simulink model "SildeModel_control_compare"  (R2022b)
settings: Solver=ode4  StartTime=0.0  StopTime=t_total  FixedStep=sim_dt  RelTol=1e-3  EnableMultiTasking=on
InitFcn:
  | InitialCondition
values from neighbouring files (symbols this model uses):
  I_B = diag([200, 250, 300])    [InitialCondition.m]
  lambda_max_J = max(eig(I_B))    [InitialCondition.m]
  mrp0 = [0.2, 0.3, -0.3]    [InitialCondition.m]
  MRP_REAL0 = MRP_REAL0'    [InitialCondition.m]
  mrpf = [0 0 0]'    [InitialCondition.m]
  sim_dt = 0.01    [InitialCondition.m]
  Tau_SEQ = [Tau_SEQ;   Tau_EXT]    [InitialCondition.m]
  w0 = w0(:)    [Gauss_opt_mrp.m]    (also in InitialCondition.m = [0; 0; 0])
settings Model: Creator=Administrator  LastModifiedBy=33592
settings DataIOCC: ExternalInput=[t, y]  LimitDataPoints=on  MaxDataPoints=15000  ReturnWorkspaceOutputs=off
settings OptimizationCC: LifeSpan=inf
settings DebuggingCC: MultiTaskCondExecSysMsg=warning  MultiTaskRateTransMsg=warning  UnconnectedInputMsg=warning  UnconnectedOutputMsg=warning  UnconnectedLineMsg=warning  AllowSymbolicDim=off  SFUnexpectedBacktrackingDiag=warning  SFNoUnconditionalDefaultTransitionDiag=warning  SFExecutionAtInitializationDiag=none  SFMachineParentedDataDiag=warning  ArithmeticOperatorsInVariantConditions=warning
settings ModelReferenceCC: EnableRefExpFcnMdlSchedulingChecks=on  PropagateSignalLabelsOutOfModel=off
settings SFSimCC: SimUseLocalCustomCode=off  CustomCodeUndefinedFunction=UseInterfaceOnly
settings RTWCC: RTWUseLocalCustomCode=off
settings CodeAppCC: StateflowObjectComments=on
settings GRTTargetCC: TargetLangStandard=C89/C90 (ANSI)
settings ConfigComp: CovMetricSettings=dw  CovSaveCumulativeToWorkspaceVar=on  CovSaveSingleToWorkspaceVar=on  CovExternalEMLEnable=off

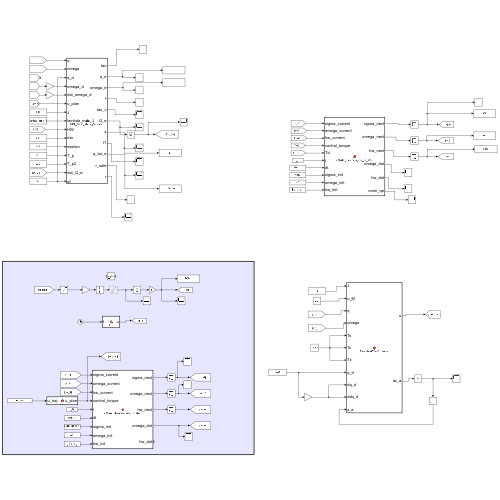
[thumbnail: Simulink's stored preview of the top-level diagram]
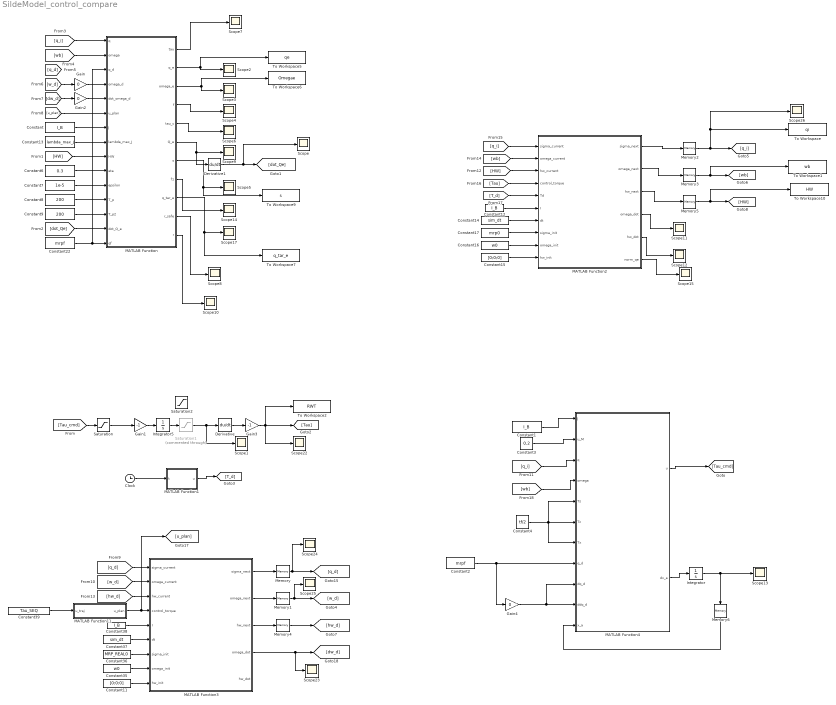
== system SildeModel_control_compare ==
  Clock : Clock
  Constant{,1,12,38} (4 alike) : Constant  Value=I_B
  Constant11 : Constant  Value=[0;0;0]
  Constant13 : Constant  Value=lambda_max_J
  Constant14 : Constant  Value=sim_dt
  Constant15 : Constant  Value=[0;0;0]
  Constant16 : Constant  Value=w0
  Constant17 : Constant  Value=mrp0
  Constant2 : Constant  Value=mrpf
  Constant22 : Constant  Value=mrpf
  Constant3 : Constant  Value=0.2
  Constant35 : Constant  Value=w0
  Constant36 : Constant  Value=MRP_REAL0
  Constant37 : Constant  Value=sim_dt
  Constant39 : Constant  Value=Tau_SEQ
  Constant4 : Constant  Value=tf/2
  Constant6 : Constant  Value=0.3
  Constant7 : Constant  Value=1e-5
  Constant8 : Constant  Value=200
  Constant9 : Constant  Value=200
  Derivative : Derivative
  Derivative1 : Derivative
  Gain : Gain  Gain=0
  Gain1 : Gain  Gain=-1
  Gain2 : Gain  Gain=0
  Gain3 : Gain  Gain=-1
  Gain4 : Gain  Gain=0
  Integrator : Integrator
  Integrator5 : Integrator
  MATLAB Function : MATLAB Function  TreatAsAtomicUnit=on
  MATLAB Function1 : MATLAB Function  TreatAsAtomicUnit=on
  MATLAB Function11 : MATLAB Function  TreatAsAtomicUnit=on
  MATLAB Function2 : MATLAB Function  TreatAsAtomicUnit=on
  MATLAB Function3 : MATLAB Function  TreatAsAtomicUnit=on
  MATLAB Function4 : MATLAB Function  TreatAsAtomicUnit=on
  Memory{,1..6} (7 alike) : Memory
  Saturation : Saturate  UpperLimit=0.2  LowerLimit=-0.2
  Saturation1 : Saturate  Commented=through  UpperLimit=4  LowerLimit=-4
  Saturation2 : Saturate  UpperLimit=4  LowerLimit=-4
  Scope{,1..15,17,22..26} (22 alike) : Scope
  To Workspace : ToWorkspace  VariableName=qi  SampleTime=-1
  To Workspace1 : ToWorkspace  VariableName=wb  SampleTime=-1
  To Workspace10 : ToWorkspace  VariableName=HW  SampleTime=-1
  To Workspace2 : ToWorkspace  VariableName=RWT  SampleTime=-1
  To Workspace5 : ToWorkspace  VariableName=qe  SampleTime=-1
  To Workspace6 : ToWorkspace  VariableName=Omegae  SampleTime=-1
  To Workspace7 : ToWorkspace  VariableName=q_tar_e  SampleTime=-1
  To Workspace9 : ToWorkspace  VariableName=s  SampleTime=-1
  wires:
  [q_i] -> MATLAB Function/1(q)
  [wb] -> MATLAB Function/2(omega)
  Constant/1 -> MATLAB Function/7(J)
  MATLAB Function/2(q_e) -> Scope2/1, To Workspace5/1
  Constant6/1 -> MATLAB Function/10(eta)
  Constant7/1 -> MATLAB Function/11(epsilon)
  Constant8/1 -> MATLAB Function/12(T_p)
  Constant9/1 -> MATLAB Function/13(T_p2)
  MATLAB Function/3(omega_e) -> Scope3/1, To Workspace6/1
  MATLAB Function/4(f) -> Scope4/1
  Constant13/1 -> MATLAB Function/8(lambda_max_J)
  MATLAB Function/7(s) -> To Workspace9/1, Scope5/1
  MATLAB Function/5(tau_c) -> Scope6/1
  MATLAB Function/6(Q_e) -> Derivative1/1, Scope9/1
  Clock/1 -> MATLAB Function1/1(t)
  MATLAB Function1/1(u) -> [T_d]
  MATLAB Function/8(f1) -> Scope14/1
  Constant22/1 -> MATLAB Function/3(q_d), MATLAB Function/15(qf)
  MATLAB Function/9(q_tar_e) -> To Workspace7/1, Scope17/1
  Gain1/1 -> Integrator5/1
  Constant35/1 -> MATLAB Function3/8(omega_init)
  Constant36/1 -> MATLAB Function3/7(sigma_init)
  Constant37/1 -> MATLAB Function3/6(dt)
  Constant38/1 -> MATLAB Function3/5(I)
  Constant39/1 -> MATLAB Function11/1(u_traj)
  MATLAB Function11/1(u_plan) -> [u_plan], MATLAB Function3/4(control_torque)
  MATLAB Function3/1(sigma_next) -> Memory/1
  Memory/1 -> [q_d], Scope24/1
  MATLAB Function3/2(omega_next) -> Memory1/1
  Memory1/1 -> [w_d], Scope25/1
  MATLAB Function3/4(omega_dot) -> Scope23/1, [dw_d]
  MATLAB Function3/3(hw_next) -> Memory4/1
  Memory4/1 -> [hw_d]
  [q_d] -> MATLAB Function3/1(sigma_current)
  [w_d] -> MATLAB Function3/2(omega_current)
  [hw_d] -> MATLAB Function3/3(hw_current)
  Constant11/1 -> MATLAB Function3/9(hw_init)
  MATLAB Function2/1(sigma_next) -> Memory2/1
  Memory3/1 -> To Workspace1/1, [wb]
  Memory2/1 -> [q_i], To Workspace/1, Scope26/1
  MATLAB Function2/2(omega_next) -> Memory3/1
  MATLAB Function2/3(hw_next) -> Memory5/1
  MATLAB Function2/4(omega_dot) -> Scope11/1
  MATLAB Function2/5(hw_dot) -> Scope12/1
  Memory5/1 -> To Workspace10/1, [HW]
  [HW] -> MATLAB Function2/3(hw_current)
  [wb] -> MATLAB Function2/2(omega_current)
  [q_i] -> MATLAB Function2/1(sigma_current)
  [Tau] -> MATLAB Function2/4(control_torque)
  [T_d] -> MATLAB Function2/5(Td)
  Constant12/1 -> MATLAB Function2/6(I)
  Constant14/1 -> MATLAB Function2/7(dt)
  Constant17/1 -> MATLAB Function2/8(sigma_init)
  Constant16/1 -> MATLAB Function2/9(omega_init)
  Constant15/1 -> MATLAB Function2/10(hw_init)
  [HW] -> MATLAB Function/9(HW)
  Derivative/1 -> Gain3/1
  Gain3/1 -> [Tau], To Workspace2/1, Scope22/1
  [u_plan] -> MATLAB Function/6(u_plan)
  [Tau_cmd] -> Saturation/1
  Saturation/1 -> Gain1/1
  Derivative1/1 -> Scope/1, [dot_Qe]
  [dot_Qe] -> MATLAB Function/14(dot_Q_e)
  MATLAB Function/10(r_safe) -> Scope8/1
  MATLAB Function/11(r) -> Scope10/1
  MATLAB Function/1(tau) -> Scope7/1
  [w_d] -> Gain/1
  [dw_d] -> Gain2/1
  Gain/1 -> MATLAB Function/4(omega_d)
  Gain2/1 -> MATLAB Function/5(dot_omega_d)
  Integrator5/1 -> Saturation1/1
  Saturation1/1 -> Scope1/1, Derivative/1
  Constant1/1 -> MATLAB Function4/1(J)
  [q_i] -> MATLAB Function4/3(q)
  [wb] -> MATLAB Function4/4(omega)
  Constant2/1 -> MATLAB Function4/8(q_d), Gain4/1
  Gain4/1 -> MATLAB Function4/9(dq_d), MATLAB Function4/10(ddq_d)
  MATLAB Function4/2(dx_a) -> Integrator/1
  Integrator/1 -> Scope13/1, Memory6/1
  Memory6/1 -> MATLAB Function4/11(x_a)
  MATLAB Function4/1(u) -> [Tau_cmd]
  Constant3/1 -> MATLAB Function4/2(u_M)
  MATLAB Function2/6(norm_qe) -> Scope15/1
  Constant4/1 -> MATLAB Function4/7(Tx), MATLAB Function4/5(Ts), MATLAB Function4/6(Tc)

== matlab function SildeModel_control_compare/MATLAB Function4 ==
  data: J input; u_M input; u output size=[3,1]; q input size=[3,1]; omega input size=[3,1]; Ts input; Tc input; Tx input; q_d input size=[3,1]; dq_d input size=[3,1]; ddq_d input size=[3,1]; x_a input size=[3,1]; dx_a output size=[3,1]
function [u, dx_a] = PrescribedTimeController(J,u_M,q, omega,Ts,Tc,Tx, q_d, dq_d, ddq_d, x_a)
    % 基于 "Distributed Prescribed-Time Attitude Coordination..." 论文设计的单航天器控制器
    % 包含预设时间收敛 (Prescribed-Time) 和 输入抗饱和 (Input Saturation)

    %% 1. 物理参数与控制器增益 (需根据实际卫星调整)
    % 惯量矩阵 [cite: 649] (示例值，请替换为真实值)
    
    

    
    % 幂次参数 (0 < v < 0.5)
    v1 = 0.1; % [cite: 242]
    v2 = 0.1; % [cite: 357]
    
    % 增益系数
    k  = 0.01;   % 滑模面增益 [cite: 235]
    k1 = 0.01;   % 控制律增益 [cite: 357]
    k2 = 40;   % 抗饱和增益 [cite: 360]
    c  = 0.01;   % 鲁棒项增益 [cite: 351]
    zeta = 0.05; % 避免抖动的平滑参数 

    %% 2. 运动学与动力学辅助计算
    % 计算 T(q) 矩阵 [cite: 83]
    q_sq = q' * q;
    I3 = eye(3);
    q_cross = [0, -q(3), q(2); q(3), 0, -q(1); -q(2), q(1), 0]; % [cite: 89]
    T_mat = 0.5 * (0.5 * (1 - q_sq) * I3 + q_cross + q * q');
    
    % 计算姿态变化率 x2 = dq (MRP rate)
    x2 = T_mat * omega; % [cite: 81]
    
    % 计算 g(x1) 及其逆矩阵
    % g(x1) = T(q) * J^-1 [cite: 100]
    g_x1 = T_mat / J; 
    g_inv = J / T_mat; % 也就是 inv(g_x1)
    
    % 计算 f(x1, x2) [cite: 94-96]
    % 为了避免复杂的 dP/dt 计算，利用等式关系: dot(x2) = f + g*u
    % 直接通过运动学微分计算 f: f = dot(T)*omega + T*J^-1*(-omega x J*omega)
    dot_q = x2;
    % dot(T) 的各项导数
    d_q_sq = 2 * q' * dot_q;
    d_q_cross = [0, -dot_q(3), dot_q(2); dot_q(3), 0, -dot_q(1); -dot_q(2), dot_q(1), 0];
    d_qqT = dot_q * q' + q * dot_q';
    dot_T_mat = 0.5 * (-0.5 * d_q_sq * I3 + d_q_cross + d_qqT);
    
    omega_cross = [0, -omega(3), omega(2); omega(3), 0, -omega(1); -omega(2), omega(1), 0];
    % 系统非线性项 f
    f_sys = dot_T_mat * omega + T_mat * (J \ (-omega_cross * J * omega));

    %% 3. 误差定义
    % 论文 Remark 1 建议使用线性差值简化设计 [cite: 102-115]
    x1_tilde = q - q_d;      % [cite: 102]
    x2_tilde = x2 - dq_d;    % [cite: 103]
    
    %% 4. 预设时间滑模面 (Sliding Surface) 设计
    % Lyapunov 函数 V_x1 [cite: 242]
    V_x1 = 0.5 * (x1_tilde' * x1_tilde);
    
    % 防止 V_x1 为 0 导致除法奇异，加极小值保护
    if V_x1 < 1e-8
        term_time_s = zeros(3,1);
        d_term_time_s = zeros(3,1);
    else
        % 预设时间项: (1/(2*v1*Ts)) * exp(V^v1) * V^-v1 * x1_tilde
        Coeff_s = (1 / (2 * v1 * Ts));
        Exp_V = exp(V_x1^v1);
        V_inv_v1 = V_x1^(-v1);
        
        term_time_s = Coeff_s * Exp_V * V_inv_v1 * x1_tilde; % [cite: 235]
        
        % 接下来计算 F 项所需的该项导数 (Chain Rule)
        % d/dt( term )
        dV_dt = x1_tilde' * x2_tilde; % V 的导数
        
        % d/dt( exp(V^v1) * V^-v1 ) 
        % = exp(...) * v1*V^(v1-1)*dV * V^-v1  +  exp(...) * (-v1)*V^(-v1-1)*dV
        % 提取公因式简化计算
        d_scalar_part = Coeff_s * Exp_V * (v1 * V_x1^(v1-1) * dV_dt * V_inv_v1 - v1 * V_x1^(-v1-1) * dV_dt);
        
        % 全导数 = 标量部分的导数 * 向量 + 标量部分 * 向量的导数
        d_term_time_s = d_scalar_part * x1_tilde + (Coeff_s * Exp_V * V_inv_v1) * x2_tilde;
    end

    % 滑模面 s [cite: 235]
    s = x2_tilde + k * x1_tilde + term_time_s;

    %% 5. 控制律计算
    % 计算 F 项 (用于抵消非线性) [cite: 278, 44]
    % F = f(x1,x2) + d/dt(其他滑模项) - ddq_d
    % 注意: 论文公式 (43) 中 dot(s) = F + g*u - dq0_dot. 
    % 这里我们把 -dq0_dot (即 -ddq_d) 包含在 F 的计算逻辑里
    F_term = f_sys - ddq_d + k * x2_tilde + d_term_time_s; 

    % 计算滑模面的 Lyapunov 函数 V_s [cite: 352]
    V_s = 0.5 * (s' * s);
    
    % 预设时间收敛项 (控制器部分)
    if V_s < 1e-8
        term_time_c = zeros(3,1);
    else
        term_time_c = (1 / (2 * v2 * Tc)) * exp(V_s^v2) * V_s^(-v2) * s; % [cite: 350]
    end
    
    % 鲁棒项 (Robust Term) [cite: 351]
    % Phi = 1 + ||q|| + ||q||^2
    Phi = 1 + norm(q) + norm(q)^2;
    robust_term = c * Phi * s / (norm(s) + zeta); % 使用 Sigmoid 近似 sign(s) 

    % 计算期望控制力矩 u (未饱和) [cite: 350]
    % u = g^-1 * ( -F - k1*s - term_time_c - robust + xa )
    u_cmd = g_inv * (-F_term - k1 * s - term_time_c - robust_term + x_a);

    %% 6. 执行器饱和与自适应补偿
    % 应用饱和函数 [cite: 87]
    u_applied = zeros(3,1);
    for i = 1:3
        u_applied(i) = sign(u_cmd(i)) * min(abs(u_cmd(i)), u_M);
    end
    
    % 输出 u
    u = u_applied;
    
    % 计算输入差值 Delta u [cite: 360]
    delta_u = u_applied - u_cmd;

    %% 7. 抗饱和自适应律更新 (Output dx_a)
    % Lyapunov 函数 V_xa [cite: 360]
    V_xa = 0.5 * (x_a' * x_a);
    
    if V_xa < 1e-8
        term_time_x = zeros(3,1);
    else
        term_time_x = (1 / (2 * v2 * Tx)) * exp(V_xa^v2) * V_xa^(-v2) * x_a; % [cite: 359]
    end
    
    % 自适应律微分方程 [cite: 359]
    dx_a = -k2 * x_a - term_time_x + g_x1 * delta_u;
    
end

== matlab function SildeModel_control_compare/MATLAB Function3 ==
  data: sigma_current input; sigma_next output; omega_current input; hw_current input; control_torque input; I input; dt input; omega_next output; hw_next output; omega_dot output; sigma_init input; omega_init input; hw_init input; hw_dot output
function [sigma_next, omega_next, hw_next, omega_dot, hw_dot] = attitude_dynamics_mrp_rw_step(...
    sigma_current, omega_current, hw_current, control_torque, I, dt, sigma_init, omega_init, hw_init)
% 单步MRP姿态动力学计算（含反作用飞轮）- 用于Simulink
% 输入:
%   sigma_current - 当前MRP [σ1, σ2, σ3] (3×1)
%   omega_current - 当前角速度 [ω1, ω2, ω3] (3×1)
%   hw_current - 当前飞轮角动量 [hw1, hw2, hw3] (3×1)
%   control_torque - 控制力矩 [u1, u2, u3] (3×1) = -ḣw
%   I - 转动惯量矩阵 (3×3)
%   dt - 时间步长
%   reset - 重置信号，当为true时使用初始值
%   sigma_init - 初始MRP [σ1, σ2, σ3] (3×1)
%   omega_init - 初始角速度 [ω1, ω2, ω3] (3×1)
%   hw_init - 初始飞轮角动量 [hw1, hw2, hw3] (3×1)
% 输出:
%   sigma_next - 下一步MRP (3×1)
%   omega_next - 下一步角速度 (3×1)
%   hw_next - 下一步飞轮角动量 (3×1)
%   omega_dot - 当前角加速度 (3×1)
%   hw_dot - 当前飞轮角动量变化率 (3×1)
%   q_out - 对应的四元数 [q1, q2, q3, q4] (4×1)，用于参考
%   is_initialized - 初始化标志

    persistent initialized;
    
    % 第一次调用时初始化persistent变量
    if isempty(initialized)
        initialized = false;
    end
    
    % MRP动力学微分方程
    function dsigma = mrp_derivative(sigma, omega)
        % MRP运动学方程: σ̇ = G(σ)ω
        sigma_sq = sigma' * sigma;
        sigma_tilde = [0, -sigma(3), sigma(2); 
                      sigma(3), 0, -sigma(1);
                      -sigma(2), sigma(1), 0];
        
        G = 0.25 * ((1 - sigma_sq) * eye(3) + 2 * sigma_tilde + 2 * (sigma * sigma'));
        dsigma = G * omega;
    end

    % 角速度动力学微分方程（含飞轮）
    function dw = angular_velocity_derivative_rw(w, hw, u, I_matrix)
        % 欧拉动力学方程（含飞轮）: Iω̇ = u - ω × (Iω + hw)
        % 其中 u = -ḣw 是飞轮控制力矩
        dw = I_matrix \ (u - cross(w, I_matrix * w + hw));
    end

    % 飞轮角动量动力学微分方程
    function dhw = wheel_momentum_derivative(u)
        % 飞轮动力学: ḣw = -u
        % 其中 u = -ḣw 是飞轮控制力矩
        dhw = -u;
    end

    % 检查是否需要切换到影子MRP
    function sigma_checked = check_shadow_mrp(sigma)
        sigma_sq = sigma' * sigma;
        if sigma_sq > 1
            % 切换到影子MRP
            sigma_checked = -sigma / sigma_sq;
        else
            sigma_checked = sigma;
        end
    end

    % 处理初始化和重置
    if ~initialized
        % 使用初始值
        current_sigma = sigma_init(:);
        current_w = omega_init(:);
        current_hw = hw_init(:);
        initialized = true;
        is_initialized = true;
    else
        % 使用当前状态
        current_sigma = sigma_current(:);
        current_w = omega_current(:);
        current_hw = hw_current(:);
        is_initialized = false;
    end
    
    current_u = control_torque(:);
    
    % 计算角加速度和飞轮角动量变化率（用于输出）
    omega_dot = angular_velocity_derivative_rw(current_w, current_hw, current_u, I);
    hw_dot = wheel_momentum_derivative(current_u);
    
    % 使用四阶龙格-库塔法进行一步积分
    % k1
    k1_sigma = mrp_derivative(current_sigma, current_w);
    k1_w = angular_velocity_derivative_rw(current_w, current_hw, current_u, I);
    k1_hw = wheel_momentum_derivative(current_u);
    
    % k2
    k2_sigma = mrp_derivative(current_sigma + 0.5 * dt * k1_sigma, current_w + 0.5 * dt * k1_w);
    k2_w = angular_velocity_derivative_rw(current_w + 0.5 * dt * k1_w, current_hw + 0.5 * dt * k1_hw, current_u, I);
    k2_hw = wheel_momentum_derivative(current_u);
    
    % k3
    k3_sigma = mrp_derivative(current_sigma + 0.5 * dt * k2_sigma, current_w + 0.5 * dt * k2_w);
    k3_w = angular_velocity_derivative_rw(current_w + 0.5 * dt * k2_w, current_hw + 0.5 * dt * k2_hw, current_u, I);
    k3_hw = wheel_momentum_derivative(current_u);
    
    % k4
    k4_sigma = mrp_derivative(current_sigma + dt * k3_sigma, current_w + dt * k3_w);
    k4_w = angular_velocity_derivative_rw(current_w + dt * k3_w, current_hw + dt * k3_hw, current_u, I);
    k4_hw = wheel_momentum_derivative(current_u);
    
    % 更新MRP、角速度和飞轮角动量
    next_sigma = current_sigma + (dt / 6) * (k1_sigma + 2*k2_sigma + 2*k3_sigma + k4_sigma);
    next_w = current_w + (dt / 6) * (k1_w + 2*k2_w + 2*k3_w + k4_w);
    next_hw = current_hw + (dt / 6) * (k1_hw + 2*k2_hw + 2*k3_hw + k4_hw);
    
    % 检查并可能切换到影子MRP
    sigma_next = check_shadow_mrp(next_sigma);
    omega_next = next_w;
    hw_next = next_hw;

end

== matlab function SildeModel_control_compare/MATLAB Function11 ==
  data: u_traj input; u_plan output
function u_plan  = fcn(u_traj)

persistent N

if isempty(N)
    N = 1;
end

u_traj = u_traj';
u_plan = u_traj(:,N);
N = N+1;

== matlab function SildeModel_control_compare/MATLAB Function1 ==
  data: t input; u output
function u = fcn(t)

% u = 0.01*[sin(2*t), cos(1*t), 1]';

u = 0.01*[sin(2*t), cos(1*t), cos(t+2)]';

== matlab function SildeModel_control_compare/MATLAB Function ==
  data: q input; omega input; q_d input; omega_d input; dot_omega_d input; u_plan input; tau output size=3; J input; lambda_max_J input; HW input; eta input; epsilon input; T_p input; T_p2 input; dot_Q_e input; q_e output size=3; omega_e output size=3; f output size=3; tau_c output size=3; Q_e output size=3; s output size=3; f1 output size=3; qf input size=3; q_tar_e output size=3; r_safe output size=1; r output size=1
function [tau, q_e, omega_e, f, tau_c, Q_e, s, f1, q_tar_e, r_safe, r] = ...
    MRP_SlidingMode_Controller(q, omega, q_d, omega_d, dot_omega_d, u_plan,J, lambda_max_J, HW, ...
                                eta, epsilon, T_p, T_p2, dot_Q_e, qf)
% MRP_SlidingMode_Controller
% 基于修正罗德里格斯参数(MRP)的预设时间滑模姿态控制器
%
% 输入:
%   q           - 当前姿态MRP (3×1)
%   q_d         - 期望姿态MRP (3×1)
%   omega       - 当前角速度 (3×1, 体坐标系)
%   omega_d     - 期望角速度 (3×1)
%   dot_omega_d - 期望角加速度 (3×1)
%   J           - 转动惯量矩阵 (3×3)
%   lambda_max_J- J的最大特征值 (标量)
%   hat_d       - 干扰估计 (3×1)
%   eta, epsilon, T_p, T_p2, a_d - 控制器参数
%
% 输出:
%   tau     - 控制力矩 (3×1)
%   q_e     - 姿态误差MRP (3×1)
%   omega_e - 角速度误差 (3×1)
%   f       - 前馈补偿项 (3×1)
%   tau_c   - 控制项 (3×1)
%   Q_e     - 滑模项函数值 (3×1)
%   s       - 滑模变量 (3×1)
%   dot_Q_e - Q_e的导数 (3×1)

%% ===== 常数计算 =====
c1 = pi / (eta * T_p);
k1 = 2^(2 + 1.5*eta);
k2 = 2^(1 - eta/2);

c2 = pi/ (eta *T_p2);
beta1 = 2^eta * (lambda_max_J/2)^(1 - eta/2);
beta2 = (lambda_max_J/2)^(1 + eta/2);

epsilon1 = 2*c1*k1*epsilon^(1-eta);


%% ===== 姿态误差与角速度误差 =====
q_e = mrp_error(q, q_d);
q_tar_e = mrp_error(q, qf);
C = mrp_to_dcm(q_e);                           % 误差DCM
omega_e = omega - C * omega_d;

%% ===== 计算 Q_e 和 s =====
r = norm(q_e);
Q_e = c1*k1*q_e / (r + epsilon)^eta + c1*k2*q_e / (r + epsilon)^(-eta);
s = omega_e + Q_e;

%% ===== 前馈补偿 f =====
f = -skew(omega)*(J*omega+HW) ...
    - J*C*dot_omega_d ...
    + J*skew(omega_e)*C*omega_d;
f1 = -skew(omega)*J*omega;

%% ===== dot_Q_e 推导实现 =====
r_safe = sqrt(q_e.' * q_e + epsilon^2);

phi  = c1*( k1*(r_safe + epsilon)^(-eta) + k2*(r_safe + epsilon)^(eta) );
dphi = c1*eta*( -k1*(r_safe + epsilon)^(-eta-1) + k2*(r_safe + epsilon)^(eta-1) );

T_q = 0.25*((1 - q_e.'*q_e)*eye(3) + 2*skew(q_e) + 2*(q_e*q_e.'));
dot_q_e = T_q * omega_e;

scalar_proj = q_e.' * dot_q_e;
dot_Q_e = phi * dot_q_e + (dphi / r_safe) * scalar_proj * q_e;
% k_s = 0.1;

%% ===== 控制律 tau_c =====
norm_s = norm(s);
% tau_c = -c2*beta1 * s / (norm_s + epsilon1)^eta ...
%         -c2*beta2 * s / (norm_s + epsilon1)^(-eta) ...
%         - J * dot_Q_e;

tau_c = -c2*beta1 * s / (norm_s + epsilon1)^eta ...
        -c2*beta2 * s / (norm_s + epsilon1)^(-eta) ...
        - J * dot_Q_e;

% for i = 1:3
%     if norm(tau_c(i)) > 0.1
%         tau_c(i) = 0.1*sign(tau_c(i));
%     end
% end

%% ===== 最终控制力矩 =====
tau = tau_c + u_plan;
% tau = f + tau_c;
% tau = +u_plan;

end

%% ===== 辅助函数 =====
function q_e = mrp_error(q, q_d)
% MRP 姿态误差
denominator = 1 + (q_d'*q_d)*(q'*q) + 2*q_d'*q;
q_e = ( q_d*(q'*q - 1) + q*(1 - q_d'*q_d) - 2*skew(q_d)*q ) / denominator;
end

function C = mrp_to_dcm(q)
% 将MRP转换为方向余弦矩阵
q_norm_sq = q' * q;
denom = (1 + q_norm_sq)^2;
C = eye(3) + (8*skew(q)^2 - 4*(1 - q_norm_sq)*skew(q)) / denom;
end

function S = skew(v)
S = [0, -v(3), v(2);
     v(3), 0, -v(1);
     -v(2), v(1), 0];
end

== matlab function SildeModel_control_compare/MATLAB Function2 ==
  settings: updateMethod=DISCRETE
  data: sigma_current input; sigma_next output; omega_current input; hw_current input; control_torque input; Td input; I input; dt input; omega_next output; hw_next output size=[3,1]; omega_dot output; sigma_init input; omega_init input; hw_init input; hw_dot output; norm_qe output
function [sigma_next, omega_next, hw_next, omega_dot, hw_dot, norm_qe] = attitude_dynamics_mrp_rw_step(...
    sigma_current, omega_current, hw_current, control_torque, Td, I, dt, sigma_init, omega_init, hw_init)
% 单步MRP姿态动力学计算（含反作用飞轮）- 用于Simulink
% 输入:
%   sigma_current - 当前MRP [σ1, σ2, σ3] (3×1)
%   omega_current - 当前角速度 [ω1, ω2, ω3] (3×1)
%   hw_current - 当前飞轮角动量 [hw1, hw2, hw3] (3×1)
%   control_torque - 控制力矩 [u1, u2, u3] (3×1) = -ḣw
%   I - 转动惯量矩阵 (3×3)
%   dt - 时间步长
%   reset - 重置信号，当为true时使用初始值
%   sigma_init - 初始MRP [σ1, σ2, σ3] (3×1)
%   omega_init - 初始角速度 [ω1, ω2, ω3] (3×1)
%   hw_init - 初始飞轮角动量 [hw1, hw2, hw3] (3×1)
% 输出:
%   sigma_next - 下一步MRP (3×1)
%   omega_next - 下一步角速度 (3×1)
%   hw_next - 下一步飞轮角动量 (3×1)
%   omega_dot - 当前角加速度 (3×1)
%   hw_dot - 当前飞轮角动量变化率 (3×1)
%   q_out - 对应的四元数 [q1, q2, q3, q4] (4×1)，用于参考
%   is_initialized - 初始化标志

    persistent initialized;
    
    % 第一次调用时初始化persistent变量
    if isempty(initialized)
        initialized = false;
    end
    
    % MRP动力学微分方程
    function dsigma = mrp_derivative(sigma, omega)
        % MRP运动学方程: σ̇ = G(σ)ω
        sigma_sq = sigma' * sigma;
        sigma_tilde = [0, -sigma(3), sigma(2); 
                      sigma(3), 0, -sigma(1);
                      -sigma(2), sigma(1), 0];
        
        G = 0.25 * ((1 - sigma_sq) * eye(3) + 2 * sigma_tilde + 2 * (sigma * sigma'));
        dsigma = G * omega;
    end

    % 角速度动力学微分方程（含飞轮）
    function dw = angular_velocity_derivative_rw(w, hw, u, Td, I_matrix)
        % 欧拉动力学方程（含飞轮）: Iω̇ = u - ω × (Iω + hw)
        % 其中 u = -ḣw 是飞轮控制力矩
        dw = I_matrix \ (u+Td - cross(w, I_matrix * w + hw));
    end

    % 飞轮角动量动力学微分方程
    function dhw = wheel_momentum_derivative(u)
        % 飞轮动力学: ḣw = -u
        % 其中 u = -ḣw 是飞轮控制力矩
        dhw = -u;
    end

    % 检查是否需要切换到影子MRP
    function sigma_checked = check_shadow_mrp(sigma)
        sigma_sq = sigma' * sigma;
        if sigma_sq > 1
            % 切换到影子MRP
            sigma_checked = -sigma / sigma_sq;
        else
            sigma_checked = sigma;
        end
    end

    % 处理初始化和重置
    if ~initialized
        % 使用初始值
        current_sigma = sigma_init(:);
        current_w = omega_init(:);
        current_hw = hw_init(:);
        initialized = true;
        is_initialized = true;
    else
        % 使用当前状态
        current_sigma = sigma_current(:);
        current_w = omega_current(:);
        current_hw = hw_current(:);
        is_initialized = false;
    end
    
    current_u = control_torque(:);
    
    % 计算角加速度和飞轮角动量变化率（用于输出）
    omega_dot = angular_velocity_derivative_rw(current_w, current_hw, current_u, Td, I);
    hw_dot = wheel_momentum_derivative(current_u);
    
    % 使用四阶龙格-库塔法进行一步积分
    % k1
    k1_sigma = mrp_derivative(current_sigma, current_w);
    k1_w = angular_velocity_derivative_rw(current_w, current_hw, current_u, Td, I);
    k1_hw = wheel_momentum_derivative(current_u);
    
    % k2
    k2_sigma = mrp_derivative(current_sigma + 0.5 * dt * k1_sigma, current_w + 0.5 * dt * k1_w);
    k2_w = angular_velocity_derivative_rw(current_w + 0.5 * dt * k1_w, current_hw + 0.5 * dt * k1_hw, current_u, Td, I);
    k2_hw = wheel_momentum_derivative(current_u);
    
    % k3
    k3_sigma = mrp_derivative(current_sigma + 0.5 * dt * k2_sigma, current_w + 0.5 * dt * k2_w);
    k3_w = angular_velocity_derivative_rw(current_w + 0.5 * dt * k2_w, current_hw + 0.5 * dt * k2_hw, current_u, Td, I);
    k3_hw = wheel_momentum_derivative(current_u);
    
    % k4
    k4_sigma = mrp_derivative(current_sigma + dt * k3_sigma, current_w + dt * k3_w);
    k4_w = angular_velocity_derivative_rw(current_w + dt * k3_w, current_hw + dt * k3_hw, current_u, Td, I);
    k4_hw = wheel_momentum_derivative(current_u);
    
    % 更新MRP、角速度和飞轮角动量
    next_sigma = current_sigma + (dt / 6) * (k1_sigma + 2*k2_sigma + 2*k3_sigma + k4_sigma);
    next_w = current_w + (dt / 6) * (k1_w + 2*k2_w + 2*k3_w + k4_w);
    next_hw = current_hw + (dt / 6) * (k1_hw + 2*k2_hw + 2*k3_hw + k4_hw);
    
    % 检查并可能切换到影子MRP
    sigma_next = check_shadow_mrp(next_sigma);
    omega_next = next_w;
    hw_next = next_hw;
    norm_qe = norm(sigma_next);

end
